simulink model "Stiff_RLC_Controller"  (R2023a)
settings: Solver=ode4  StartTime=0.0  StopTime=2  FixedStep=0.0005  RelTol=1e-3
settings Model: Creator=Fasih  LastModifiedBy=Fasih

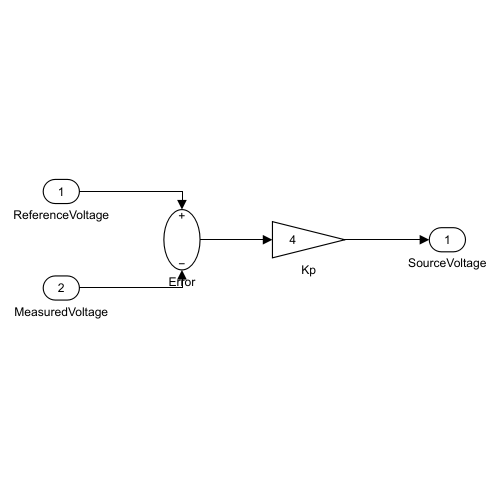
[thumbnail: Simulink's stored preview of the top-level diagram]
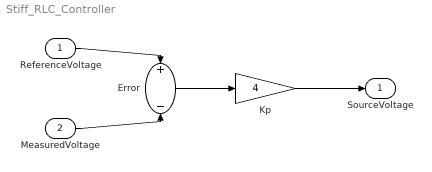
== system Stiff_RLC_Controller ==
  ReferenceVoltage : Inport
  MeasuredVoltage : Inport  Port=2
  Error : Sum  Inputs=+-
  Kp : Gain  Gain=4
  SourceVoltage : Outport
  wires:
  ReferenceVoltage/1 -> Error/1
  MeasuredVoltage/1 -> Error/2
  Error/1 -> Kp/1
  Kp/1 -> SourceVoltage/1
